simulink model "Assignment2_dcm_2021a"  (R2021a)
settings: Solver=FixedStepAuto  StartTime=0.0  StopTime=inf  FixedStep=1e-3  RelTol=1e-3  EnableMultiTasking=on
undefined symbols (not defined in the file): A0, A1, D0, D1, D10, D11, D12, D13, D2, D3, D4, D5, D6, D7, D8, D9, PTA0, PTA1, PTA2, PTB2, PTB23, PTB3, PTB9, PTC16, PTC17, PTC2, PTC3, PTC4, PTD0, PTD1, PTD2, PTD3
libraries: frdmk64flib x19, etargetslib x10
settings Model: ExtModeTrigDuration=5  Creator=MSI_NB  LastModifiedBy=xxx
settings OptimizationCC: EnhancedBackFolding=on  PassReuseOutputArgsAs=Individual arguments  ZeroExternalMemoryAtStartup=off  ZeroInternalMemoryAtStartup=off  MaxStackSize=64  OptimizeBlockOrder=speed  DifferentSizesBufferReuse=on  OptimizationCustomize=off  EfficientTunableParamExpr=on
settings DebuggingCC: ParameterTunabilityLossMsg=error
settings HardwareCC: ProdBitPerPointer=32  ProdBitPerSizeT=32  ProdBitPerPtrDiffT=32  ProdLargestAtomicInteger=Long  ProdLargestAtomicFloat=Double  ProdWordSize=32  ProdHWDeviceType=ARM Compatible->ARM Cortex
settings SFSimCC: MATLABDynamicMemAlloc=off
settings RTWCC: SystemTargetFile=ert.tlc  HardwareBoard=NXP FRDM-K64F  TLCOptions="-aInlineSetEventsForThisBaseRateFcn=TLC_FALSE -aSuppressMultiTaskScheduler=TLC_FALSE  -aRateBasedStepFcn=0"  TemplateMakefile=ert_default_tmf  Toolchain=GNU Tools for ARM Embedded Processors
settings CodeAppCC: ForceParamTrailComments=on  IgnoreCustomStorageClasses=off  OperatorAnnotations=on  SimulinkDataObjDesc=on  SFDataObjDesc=on  InsertBlockDesc=on
settings ERTTargetCC: ExtModeTransport=4  ExtModeMexFile=sendToCommService

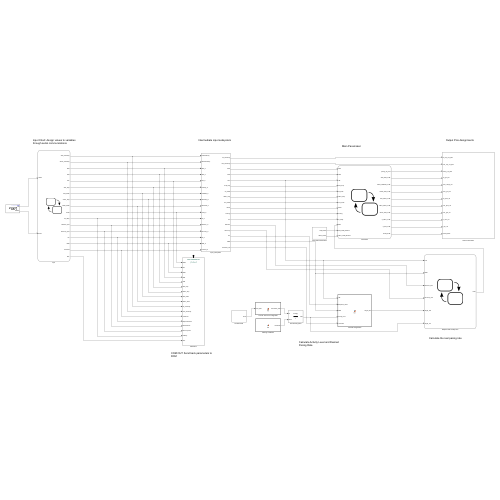
[thumbnail: Simulink's stored preview of the top-level diagram]
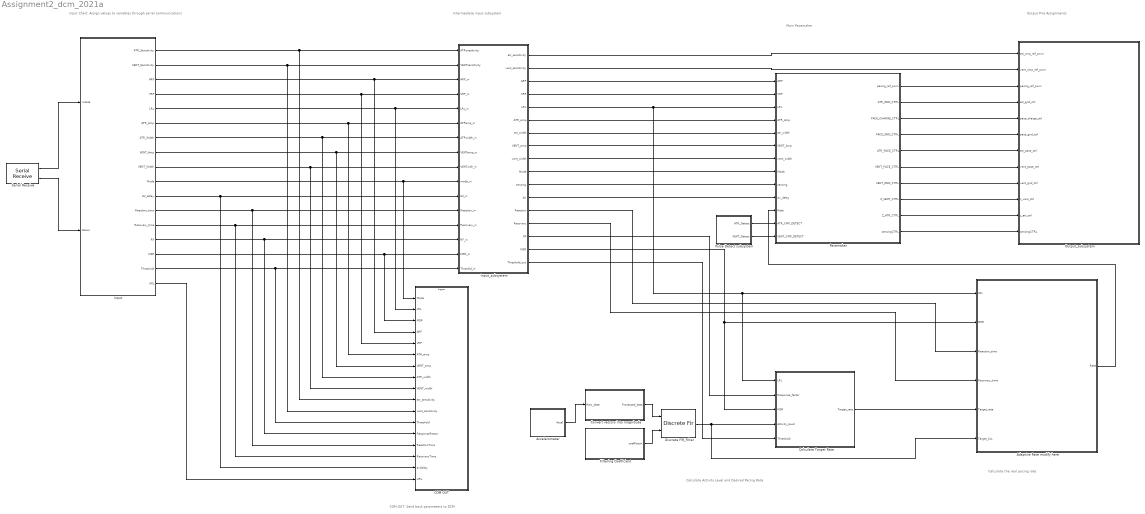
== system Assignment2_dcm_2021a ==
  note: Input Chart: Assign values to variables through serial communications
  note: COM OUT: Send back parameters to DCM
  note: Calculate Activity Level and Desired Pacing Rate
  note: Calculate the real pacing rate
  note: Output Pins Assignments
  note: Main Pacemaker
  note: Intermediate input subsystem
  Accelerometer : Subsystem
  Adaptive Rate modify here : Stateflow chart  TreatAsAtomicUnit=on
      settings: PortSchema="{\"entries\":[{\"content\":{\"sides\":[{\"content\":{\"connectorIds\":[\"In6\",\"In5\",\"In1\",\"In2\",\"In4\",\"In3\"]},\"type\":\"ConnectorPlacement.EquallySpacedRectSide\",\"uuid\":\"39a759a2-6776-4dc2-bf13-d3cf12be31b7\"},{\"content\":{\"connectorIds\":[\"Out1\"],\"side\":\"RIGHT\"},\"type\":\"ConnectorPlacement.EquallySpacedRectSide\",\"uuid\":\"311af287-9fec-40a9-86fa-7b14c4c20eba\"},{\"content\":{\"connectorIds\":[],\"side\":\"TOP\"},\"type\":\"ConnectorPlacement.EquallySpacedRectSide\",\"uuid\":\"bb2111ef-c928-45d1-9471-772f70406d6d\"}]},\"type\":\"ConnectorPlacement.EquallySpacedConnector\",\"uuid\":\"d6adbde0-79db-4fc2-a399-102b42b2f3be\"}],\"packageUris\":[\"http://schema.mathworks.com/mf0/Connector/R2020b\"],\"version\":\"1.0\"}"
  COM OUT : Subsystem  TreatAsAtomicUnit=on
  Calculate Target Rate : MATLAB Function  TreatAsAtomicUnit=on
  Convert vectors into magnitude : MATLAB Function  TreatAsAtomicUnit=on
  Discrete FIR_Filter : DiscreteFir  CoefSource=Input port  Coefficients=[0.05, 0.05, 0.05, 0.05, 0.05, 0.05, 0.05, 0.05, 0.05, 0.05, 0.05, 0.05, 0.05, 0.05, 0.05, 0.05, 0.05, 0.05, 0.05, 0.05]  SampleTime=0.01
      settings: InputPortMap=u0,u1
  Filtering Coefficient : MATLAB Function  TreatAsAtomicUnit=on
  Input : Stateflow chart  TreatAsAtomicUnit=on
      settings: PortSchema="{\"entries\":[{\"content\":{\"sides\":[{\"content\":{\"connectorIds\":[\"In1\",\"In2\"]},\"type\":\"ConnectorPlacement.EquallySpacedRectSide\",\"uuid\":\"ee3611de-e013-4c9d-af16-b184b46b299a\"},{\"content\":{\"connectorIds\":[\"Out6\",\"Out13\",\"Out1\",\"Out2\",\"Out3\",\"Out5\",\"Out7\",\"Out12\",\"Out14\",\"Out8\",\"Out15\",\"Out10\",\"Out11\",\"Out9\",\"Out4\",\"Out17\",\"Out16\"],\"side\":\"RIGHT\"},\"type\":\"ConnectorPlacement.EquallySpacedRectSide\",\"uuid\":\"205a7e36-44cf-418f-ba3c-405c0f3a2ab0\"},{\"content\":{\"connectorIds\":[],\"side\":\"TOP\"},\"type\":\"ConnectorPlacement.EquallySpacedRectSide\",\"uuid\":\"6ab59ebe-c7e2-4512-b8ce-c3a29cac6f4f\"}]},\"type\":\"ConnectorPlacement.EquallySpacedConnector\",\"uuid\":\"f4485e1d-0176-43db-b1e3-40045324a3f2\"}],\"packageUris\":[\"http://schema.mathworks.com/mf0/Connector/R2020b\"],\"version\":\"1.0\"}"
  Input_subsystem : Subsystem
  Output_subsystem : Subsystem
  Pacemaker : Stateflow chart  TreatAsAtomicUnit=on
      settings: PortSchema="{\"entries\":[{\"content\":{\"sides\":[{\"content\":{\"connectorIds\":[\"In1\",\"In10\",\"In6\",\"In8\",\"In11\",\"In7\",\"In12\",\"In3\",\"In5\",\"In13\",\"In9\",\"In2\",\"In4\"]},\"type\":\"ConnectorPlacement.EquallySpacedRectSide\",\"uuid\":\"2ef21990-d536-4d68-b59e-2b2ea3a8851a\"},{\"content\":{\"connectorIds\":[\"Out10\",\"Out1\",\"Out3\",\"Out4\",\"Out2\",\"Out6\",\"Out5\",\"Out7\",\"Out8\",\"Out9\"],\"side\":\"RIGHT\"},\"type\":\"ConnectorPlacement.EquallySpacedRectSide\",\"uuid\":\"f7b17b6e-2681-486a-8f68-6cf7f9b59642\"},{\"content\":{\"connectorIds\":[],\"side\":\"TOP\"},\"type\":\"ConnectorPlacement.EquallySpacedRectSide\",\"uuid\":\"48d212d0-9916-482c-b6c3-a579a81f1368\"},{\"content\":{\"connectorIds\":[],\"side\":\"BOTTOM\"},\"type\":\"ConnectorPlacement.EquallySpacedRectSide\",\"uuid\":\"9c2cce1f-edc0-4859-9c72-07093d7dd567\"}]},\"type\":\"ConnectorPlacement.EquallySpacedConnector\",\"uuid\":\"8d012c1f-5b6f-45ee-bba7-5808d4a194ab\"}],\"packageUris\":[\"http://schema.mathworks.com/mf0/Connector/R2020b\"],\"version\":\"1.0\"}"
  Pulse Detect subsystem : Subsystem
  Serial Receive : frdmk64flib/Serial Receive  SCIModule=0  Baudrate=uint32(9600)  Parity=None  StopBits=1  HardwareFlowControl=None  ByteOrder=LittleEndian  DataType=uint8  DataLength=37  BlockingMode=off  OutputStatus=on  SampleTime=-1
  wires:
  Pulse Detect subsystem/1(ATR_Detect) -> Pacemaker/2(ATR_CMP_DETECT)
  Pulse Detect subsystem/2(VENT_Detect) -> Pacemaker/4(VENT_CMP_DETECT)
  Pacemaker/7(Z_VENT_CTRL) -> Output_subsystem/10(" z_vent_ctrl")
  Pacemaker/8(Z_ATR_CTRL) -> Output_subsystem/11(z_atr_ctrl)
  Pacemaker/5(VENT_GND_CTRL) -> Output_subsystem/9(vent_gnd_ctrl)
  Pacemaker/2(ATR_PACE_CTRL) -> Output_subsystem/7(atr_pace_ctrl)
  Pacemaker/6(VENT_PACE_CTRL) -> Output_subsystem/8(vent_pace_ctrl)
  Pacemaker/4(PACE_GND_CTRL) -> Output_subsystem/6(pace_gnd_ctrl)
  Pacemaker/9(sensingCTRL) -> Output_subsystem/12(sensingCTRL)
  Pacemaker/3(PACE_CHARGE_CTRL) -> Output_subsystem/5(pace_charge_ctrl)
  Pacemaker/1(ATR_GND_CTRL) -> Output_subsystem/4(atr_gnd_ctrl)
  Input_subsystem/4(VRP) -> Pacemaker/10(VRP)
  Input_subsystem/3(ARP) -> Pacemaker/1(ARP)
  Input_subsystem/6(ATR_amp) -> Pacemaker/8(ATR_Amp)
  Input_subsystem/7(atr_width) -> Pacemaker/11(atr_width)
  Input_subsystem/8(VENT_amp) -> Pacemaker/7(VENT_Amp)
  Input_subsystem/9(vent_width) -> Pacemaker/12(vent_width)
  Input_subsystem/10(Mode) -> Pacemaker/3(Mode)
  Adaptive Rate modify here/1(Rate) -> Pacemaker/9(Rate)
  Input_subsystem/13(Reaction) -> Adaptive Rate modify here/1(Reaction_time)
  Input_subsystem/14(Recovery) -> Adaptive Rate modify here/2(Recovery_time)
  Pacemaker/10(pacing_ref_pwm) -> Output_subsystem/3(pacing_ref_pwm)
  Input_subsystem/2(vent_sensitivity) -> Output_subsystem/2(vent_cmp_ref_pwm)
  Input_subsystem/1(atr_sensitivity) -> Output_subsystem/1(atr_cmp_ref_pwm)
  Input_subsystem/11(sensing) -> Pacemaker/5(sensing)
  Convert vectors into magnitude/1(Processed_data) -> Discrete FIR_Filter/1
  Filtering Coefficient/1(coefficient) -> Discrete FIR_Filter/2
  Input_subsystem/16(MSR) -> Adaptive Rate modify here/5(MSR), Calculate Target Rate/3(MSR)
  Calculate Target Rate/1(Target_rate) -> Adaptive Rate modify here/4(Target_rate)
  Input_subsystem/15(RF) -> Calculate Target Rate/2(Response_factor)
  Input_subsystem/5(LRL) -> Adaptive Rate modify here/6(LRL), Calculate Target Rate/1(LRL), Pacemaker/6(LRL)
  Input_subsystem/12(AV) -> Pacemaker/13(av_delay)
  Accelerometer/1(Accel) -> Convert vectors into magnitude/1(Raw_data)
  Serial Receive/1 -> Input/1(rxdata)
  Serial Receive/2 -> Input/2(status)
  Input_subsystem/17(Threshold_out) -> Calculate Target Rate/5(Threshold)
  Discrete FIR_Filter/1 -> Adaptive Rate modify here/3(Target_LVL), Calculate Target Rate/4(Activity_level)
  Input/6(ATR_Sensitivity) -> COM OUT/10(atr_sensitivity), Input_subsystem/1(ATRsnesitivity)
  Input/13(VENT_Sensitivity) -> COM OUT/11(vent_sensitivity), Input_subsystem/2(VENTsensitivity)
  Input/1(ARP) -> COM OUT/4(ARP), Input_subsystem/3(ARP_in)
  Input/2(VRP) -> COM OUT/5(VRP), Input_subsystem/4(VRP_in)
  Input/3(LRL) -> COM OUT/2(LRL), Input_subsystem/5(LRL_in)
  Input/5(ATR_Amp) -> COM OUT/6(ATR_amp), Input_subsystem/6(ATPamp_in)
  Input/7(ATR_Width) -> COM OUT/8(ATR_width), Input_subsystem/7(ATRwidth_in)
  Input/12(VENT_Amp) -> COM OUT/7(VENT_amp), Input_subsystem/8(VENTamp_in)
  Input/14(VENT_Width) -> COM OUT/9(VENT_width), Input_subsystem/9(VENTwith_in)
  Input/8(Mode) -> COM OUT/1(Mode), Input_subsystem/10(mode_in)
  Input/15(AV_delay) -> COM OUT/16(avDelay), Input_subsystem/11(AV_in)
  Input/10(Reaction_time) -> COM OUT/14(ReactionTime), Input_subsystem/12(Reaction_in)
  Input/11(Recovery_time) -> COM OUT/15(RecoveryTime), Input_subsystem/13(Recovery_in)
  Input/9(RF) -> COM OUT/13(ResponseFactor), Input_subsystem/14(RF_in)
  Input/4(MSR) -> COM OUT/3(MSR), Input_subsystem/15(MSR_in)
  Input/17(Threshold) -> COM OUT/12(Threshold), Input_subsystem/16(Threshld_in)
  Input/16(URL) -> COM OUT/17(URL)

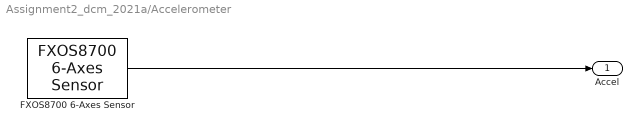
== system Assignment2_dcm_2021a/Accelerometer ==
  FXOS8700 6-Axes Sensor : frdmk64flib/FXOS8700 6-Axes Sensor  Activesensor=Accelerometer only  ODR=800Hz  HybridODR=400Hz  Accelfullrange=-4g to +4g  SampleTime=0.01
  Accel : Outport
  wires:
  FXOS8700 6-Axes Sensor/1 -> Accel/1

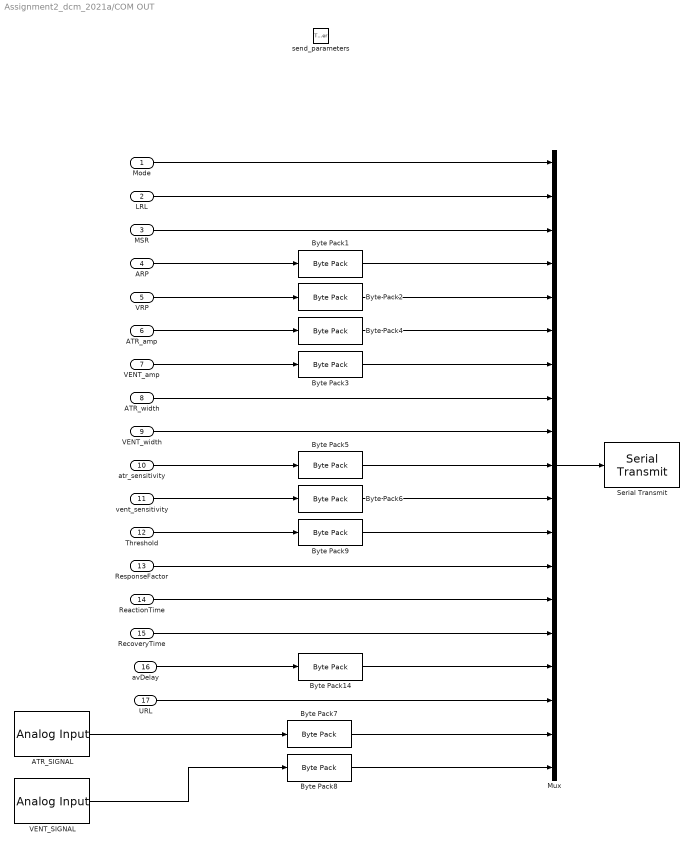
== system Assignment2_dcm_2021a/COM OUT ==
  Mode : Inport  OutDataTypeStr=uint8
  LRL : Inport  Port=2  OutDataTypeStr=uint8
  MSR : Inport  Port=3  OutDataTypeStr=uint8
  ARP : Inport  Port=4  OutDataTypeStr=uint16
  VRP : Inport  Port=5  OutDataTypeStr=uint16
  ATR_amp : Inport  Port=6  OutDataTypeStr=single
  VENT_amp : Inport  Port=7  OutDataTypeStr=single
  ATR_width : Inport  Port=8  OutDataTypeStr=uint8
  VENT_width : Inport  Port=9  OutDataTypeStr=uint8
  atr_sensitivity : Inport  Port=10  OutDataTypeStr=single
  vent_sensitivity : Inport  Port=11  OutDataTypeStr=single
  Threshold : Inport  Port=12  OutDataTypeStr=single
  ResponseFactor : Inport  Port=13  OutDataTypeStr=uint8
  ReactionTime : Inport  Port=14  OutDataTypeStr=uint8
  RecoveryTime : Inport  Port=15  OutDataTypeStr=uint8
  avDelay : Inport  Port=16  OutDataTypeStr=uint16
  URL : Inport  Port=17  OutDataTypeStr=uint8
  send_parameters : TriggerPort  TriggerType=function-call  IsSimulinkFunction=on  FunctionName=send_parameters  VariantControl=(inherit)
  ATR_SIGNAL : frdmk64flib/Analog Input  Whichpin=PTB2 (A0)  SampleTime=-1
  Byte Pack1 : etargetslib/Byte Pack  datatypes={'uint16'}  byteAlign=1
  Byte Pack14 : etargetslib/Byte Pack  datatypes={'uint16'}  byteAlign=1
  Byte Pack2 : etargetslib/Byte Pack  datatypes={'uint16'}  byteAlign=1
  Byte Pack{3..6,9} (5 alike) : etargetslib/Byte Pack  datatypes={'single'}  byteAlign=1
  Byte Pack7 : etargetslib/Byte Pack  datatypes={'double'}  byteAlign=1
  Byte Pack8 : etargetslib/Byte Pack  datatypes={'double'}  byteAlign=1
  Mux : Mux  Inputs=19
  Serial Transmit : frdmk64flib/Serial Transmit  SCIModule=0  Baudrate=uint32(9600)  Parity=None  StopBits=1  HardwareFlowControl=None  ByteOrder=LittleEndian  BlockingMode=on  OutputStatus=off
  VENT_SIGNAL : frdmk64flib/Analog Input  Whichpin=PTB3 (A1)  SampleTime=-1
  wires:
  ReactionTime/1 -> Mux/14
  avDelay/1 -> Byte Pack14/1
  VENT_width/1 -> Mux/9
  vent_sensitivity/1 -> Byte Pack6/1
  MSR/1 -> Mux/3
  VENT_amp/1 -> Byte Pack3/1
  ResponseFactor/1 -> Mux/13
  LRL/1 -> Mux/2
  VRP/1 -> Byte Pack2/1
  Byte Pack5/1 -> Mux/10
  Byte Pack3/1 -> Mux/7
  Byte Pack4/1 -> Mux/6
  ATR_amp/1 -> Byte Pack4/1
  Threshold/1 -> Byte Pack9/1
  atr_sensitivity/1 -> Byte Pack5/1
  Byte Pack2/1 -> Mux/5
  RecoveryTime/1 -> Mux/15
  Byte Pack14/1 -> Mux/16
  Mode/1 -> Mux/1
  Byte Pack9/1 -> Mux/12
  ARP/1 -> Byte Pack1/1
  URL/1 -> Mux/17
  ATR_width/1 -> Mux/8
  Byte Pack6/1 -> Mux/11
  Byte Pack1/1 -> Mux/4
  ATR_SIGNAL/1 -> Byte Pack7/1
  Byte Pack7/1 -> Mux/18
  Byte Pack8/1 -> Mux/19
  VENT_SIGNAL/1 -> Byte Pack8/1
  Mux/1 -> Serial Transmit/1

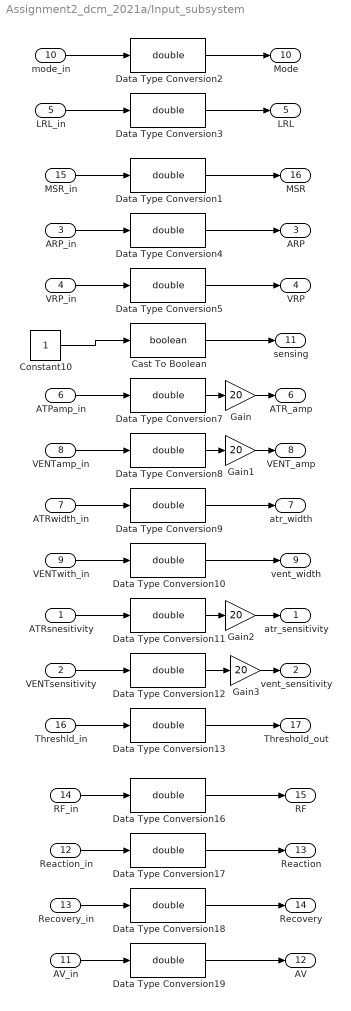
== system Assignment2_dcm_2021a/Input_subsystem ==
  ATRsnesitivity : Inport  Unit=ms
  VENTsensitivity : Inport  Port=2  Unit=ms
  ARP_in : Inport  Port=3  Unit=ms
  VRP_in : Inport  Port=4  Unit=ms
  LRL_in : Inport  Port=5  Unit=ms
  ATPamp_in : Inport  Port=6  Unit=ms
  ATRwidth_in : Inport  Port=7  Unit=ms
  VENTamp_in : Inport  Port=8  Unit=ms
  VENTwith_in : Inport  Port=9  Unit=ms
  mode_in : Inport  Port=10  Unit=ms
  AV_in : Inport  Port=11  Unit=ms
  Reaction_in : Inport  Port=12  Unit=ms
  Recovery_in : Inport  Port=13  Unit=ms
  RF_in : Inport  Port=14  Unit=ms
  MSR_in : Inport  Port=15  Unit=ms
  Threshld_in : Inport  Port=16  Unit=ms
  Cast To Boolean : DataTypeConversion  OutDataTypeStr=boolean
  Constant10 : Constant
  Data Type Conversion{1..5,7..13,16..19} (16 alike) : DataTypeConversion  OutDataTypeStr=double
  Gain{,1..3} (4 alike) : Gain  Gain=20
  atr_sensitivity : Outport
  vent_sensitivity : Outport  Port=2
  ARP : Outport  Port=3
  VRP : Outport  Port=4
  LRL : Outport  Port=5
  ATR_amp : Outport  Port=6
  atr_width : Outport  Port=7
  VENT_amp : Outport  Port=8
  vent_width : Outport  Port=9
  Mode : Outport  Port=10
  sensing : Outport  Port=11
  AV : Outport  Port=12
  Reaction : Outport  Port=13
  Recovery : Outport  Port=14
  RF : Outport  Port=15
  MSR : Outport  Port=16
  Threshold_out : Outport  Port=17
  wires:
  mode_in/1 -> Data Type Conversion2/1
  LRL_in/1 -> Data Type Conversion3/1
  MSR_in/1 -> Data Type Conversion1/1
  ARP_in/1 -> Data Type Conversion4/1
  VRP_in/1 -> Data Type Conversion5/1
  ATPamp_in/1 -> Data Type Conversion7/1
  VENTamp_in/1 -> Data Type Conversion8/1
  ATRwidth_in/1 -> Data Type Conversion9/1
  VENTwith_in/1 -> Data Type Conversion10/1
  ATRsnesitivity/1 -> Data Type Conversion11/1
  VENTsensitivity/1 -> Data Type Conversion12/1
  Threshld_in/1 -> Data Type Conversion13/1
  RF_in/1 -> Data Type Conversion16/1
  Reaction_in/1 -> Data Type Conversion17/1
  Recovery_in/1 -> Data Type Conversion18/1
  AV_in/1 -> Data Type Conversion19/1
  Data Type Conversion3/1 -> LRL/1
  Data Type Conversion1/1 -> MSR/1
  Data Type Conversion4/1 -> ARP/1
  Data Type Conversion5/1 -> VRP/1
  Cast To Boolean/1 -> sensing/1
  Data Type Conversion7/1 -> Gain/1
  Data Type Conversion8/1 -> Gain1/1
  Data Type Conversion9/1 -> atr_width/1
  Data Type Conversion10/1 -> vent_width/1
  Data Type Conversion11/1 -> Gain2/1
  Data Type Conversion12/1 -> Gain3/1
  Data Type Conversion13/1 -> Threshold_out/1
  Data Type Conversion16/1 -> RF/1
  Data Type Conversion17/1 -> Reaction/1
  Data Type Conversion18/1 -> Recovery/1
  Data Type Conversion19/1 -> AV/1
  Data Type Conversion2/1 -> Mode/1
  Constant10/1 -> Cast To Boolean/1
  Gain/1 -> ATR_amp/1
  Gain1/1 -> VENT_amp/1
  Gain2/1 -> atr_sensitivity/1
  Gain3/1 -> vent_sensitivity/1

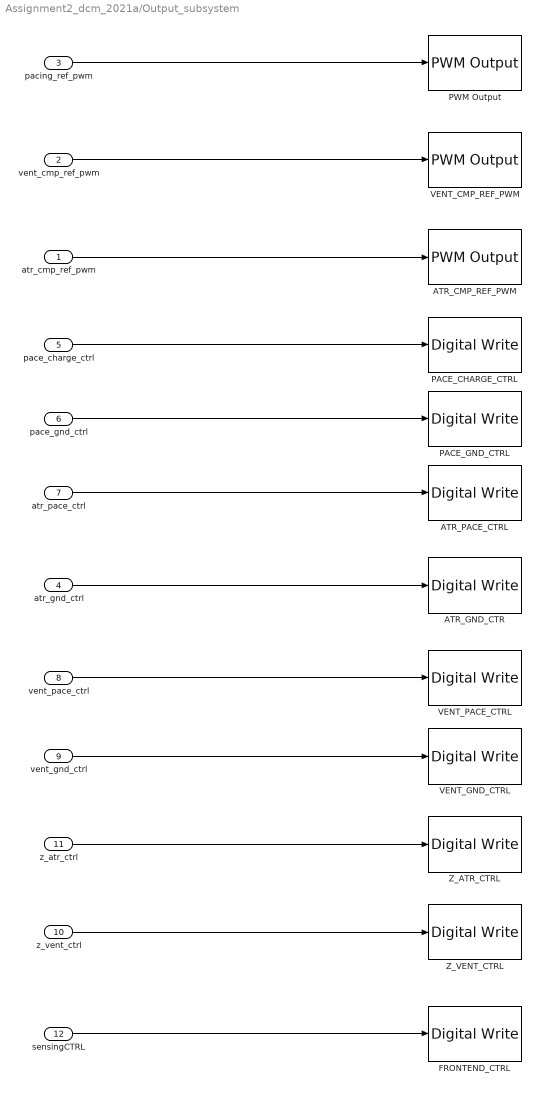
== system Assignment2_dcm_2021a/Output_subsystem ==
  atr_cmp_ref_pwm : Inport
  vent_cmp_ref_pwm : Inport  Port=2
  pacing_ref_pwm : Inport  Port=3
  atr_gnd_ctrl : Inport  Port=4
  pace_charge_ctrl : Inport  Port=5
  pace_gnd_ctrl : Inport  Port=6
  atr_pace_ctrl : Inport  Port=7
  vent_pace_ctrl : Inport  Port=8
  vent_gnd_ctrl : Inport  Port=9
  " z_vent_ctrl" : Inport  Port=10
  z_atr_ctrl : Inport  Port=11
  sensingCTRL : Inport  Port=12
  ATR_CMP_REF_PWM : frdmk64flib/PWM Output  Whichpin=PTC2 (D6)  InitialFrequency=2000  InitialDutyCycle=50
  ATR_GND_CTR : frdmk64flib/Digital Write  Whichpin=PTD2 (D11)
  ATR_PACE_CTRL : frdmk64flib/Digital Write  Whichpin=PTA0 (D8)
  FRONTEND_CTRL : frdmk64flib/Digital Write  Whichpin=PTD1 (D13)
  PACE_CHARGE_CTRL : frdmk64flib/Digital Write  Whichpin=PTB9 (D2)
  PACE_GND_CTRL : frdmk64flib/Digital Write  Whichpin=PTD0 (D10)
  PWM Output : frdmk64flib/PWM Output  Whichpin=PTA2 (D5)  InitialFrequency=2000  InitialDutyCycle=50
  VENT_CMP_REF_PWM : frdmk64flib/PWM Output  Whichpin=PTA1 (D3)  InitialFrequency=2000  InitialDutyCycle=50
  VENT_GND_CTRL : frdmk64flib/Digital Write  Whichpin=PTD3 (D12)
  VENT_PACE_CTRL : frdmk64flib/Digital Write  Whichpin=PTC4 (D9)
  Z_ATR_CTRL : frdmk64flib/Digital Write  Whichpin=PTB23 (D4)
  Z_VENT_CTRL : frdmk64flib/Digital Write  Whichpin=PTC3 (D7)
  wires:
  pace_gnd_ctrl/1 -> PACE_GND_CTRL/1
  atr_pace_ctrl/1 -> ATR_PACE_CTRL/1
  pace_charge_ctrl/1 -> PACE_CHARGE_CTRL/1
  atr_gnd_ctrl/1 -> ATR_GND_CTR/1
  vent_pace_ctrl/1 -> VENT_PACE_CTRL/1
  vent_gnd_ctrl/1 -> VENT_GND_CTRL/1
  z_atr_ctrl/1 -> Z_ATR_CTRL/1
  " z_vent_ctrl"/1 -> Z_VENT_CTRL/1
  sensingCTRL/1 -> FRONTEND_CTRL/1
  pacing_ref_pwm/1 -> PWM Output/1
  vent_cmp_ref_pwm/1 -> VENT_CMP_REF_PWM/1
  atr_cmp_ref_pwm/1 -> ATR_CMP_REF_PWM/1

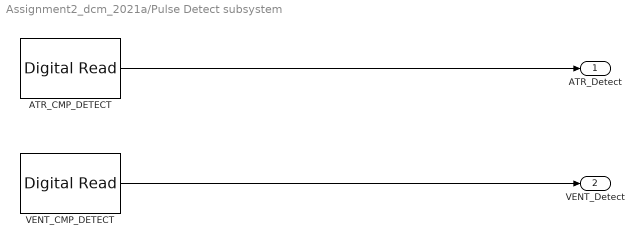
== system Assignment2_dcm_2021a/Pulse Detect subsystem ==
  ATR_CMP_DETECT : frdmk64flib/Digital Read  Whichpin=PTC16 (D0)  SampleTime=-1
  VENT_CMP_DETECT : frdmk64flib/Digital Read  Whichpin=PTC17 (D1)  SampleTime=-1
  ATR_Detect : Outport  OutDataTypeStr=boolean
  VENT_Detect : Outport  Port=2  OutDataTypeStr=boolean
  wires:
  ATR_CMP_DETECT/1 -> ATR_Detect/1
  VENT_CMP_DETECT/1 -> VENT_Detect/1

== stateflow chart Assignment2_dcm_2021a/Input ==
  settings: executeAtInitialization=1
  state SET_PARAM
    entry:
    Mode = rxdata(3);
    LRL = rxdata(4);
    MSR = rxdata(5);
    ARP =  typecast(rxdata(6:7), 'uint16');
    VRP = typecast(rxdata(8:9), 'uint16');
    ATR_Amp = typecast(rxdata(10:13),'single');
    VENT_Amp = typecast(rxdata(14:17),'single');
    ATR_Width = rxdata(18);
    VENT_Width = rxdata(19);
    ATR_Sensitivity = typecast(rxdata(20:23), 'single');
    VENT_Sensitivity = typecast(rxdata(24:27), 'single');
    Threshold = typecast(rxdata(28:31), 'single');
    RF =rxdata(32);
    Reaction_time = rxdata(33);
    Recovery_time =rxdata(34);
    AV_delay = typecast(rxdata(35:36), 'uint16');
    URL = rxdata(37);
  state Initialize
    entry:
    Mode = 1; %select mode:1-10
    LRL = 60; %ppm
    MSR = 160; %ppm
    ARP = 250; %msec
    VRP = 250; %msec
    ATR_Amp = 3.3; %Volt, will convert to dutycycle later
    VENT_Amp = 3.3; %Volt, will convert to dutycycle later
    ATR_Width = 10; %msec
    VENT_Width = 10; %msec
    ATR_Sensitivity = 3; %Volt, will convert to dutycycle later
    VENT_Sensitivity = 3; %Volt, will convert to dutycycle later
    Threshold = 1.1; %Threshold for activity level
    RF = 16; % Response Factor: 1-16
    Reaction_time = 10; %sec
    Recovery_time = 30; %sec
    AV_delay = 150;%msec
    URL = 160; %ppm
  state STANDBY
    %Waiting for COM
  state ECHO_PARAMETERS
    entry:
    send_parameters();
  SET_PARAM -> STANDBY
  (default) -> Initialize
  (junction 115) -> SET_PARAM [order 1] : [rxdata(2) == hex2dec('55')]
  STANDBY -> (junction 118) : [status==0]
  (junction 118) -> (junction 115) : [rxdata(1) == hex2dec('16')]
  Initialize -> STANDBY
  (junction 115) -> ECHO_PARAMETERS [order 2] : [rxdata(2) == hex2dec('22')]
  ECHO_PARAMETERS -> STANDBY
  data: ARP output uint16; VRP output uint16; LRL output uint8; MSR output uint8; ATR_Amp output single; ATR_Sensitivity output single; ATR_Width output uint8; Mode output uint8; RF output uint8; Reaction_time output uint8; Recovery_time output uint8; VENT_Amp output single; VENT_Sensitivity output single; VENT_Width output uint8; AV_delay output uint16; rxdata input uint8; status input uint8 size=[1 1]; URL output uint8; Threshold output single

== stateflow chart Assignment2_dcm_2021a/Pacemaker ==
  state VOO
    state Charging_Discharging
      entry:
      pacing_ref_pwm = VENT_Amp;
      pacing_period = (60000/LRL);
      ATR_PACE_CTRL = false;
      ATR_GND_CTRL = false;
      VENT_PACE_CTRL = false;
      VENT_GND_CTRL = true;
      PACE_GND_CTRL = true;
      Z_ATR_CTRL = false;
      Z_VENT_CTRL = false;
      PACE_CHARGE_CTRL = true;
    state Pacing
      entry:
      PACE_CHARGE_CTRL = false;
      ATR_PACE_CTRL = false;
      ATR_GND_CTRL = false;
      VENT_PACE_CTRL = true;
      VENT_GND_CTRL = false;
      PACE_GND_CTRL = true;
      Z_ATR_CTRL = false;
      Z_VENT_CTRL = false;
    (default) -> VOO.Charging_Discharging
    VOO.Charging_Discharging -> VOO.Pacing : after((pacing_period-vent_width),msec)
    VOO.Pacing -> VOO.Charging_Discharging : after(vent_width,msec)
  state VVI
    state Charging_Discharging
      entry:
      pacing_ref_pwm = VENT_Amp;
      pacing_period = (60000/LRL);
      sensingCTRL = sensing;
      ATR_PACE_CTRL = false;
      ATR_GND_CTRL = false;
      VENT_PACE_CTRL = false;
      VENT_GND_CTRL = true;
      PACE_GND_CTRL = true;
      Z_ATR_CTRL = false;
      Z_VENT_CTRL = false;
      PACE_CHARGE_CTRL = true;
    state Pacing
      entry:
      ATR_PACE_CTRL = false;
      ATR_GND_CTRL = false;
      VENT_PACE_CTRL = true;
      VENT_GND_CTRL = false;
      PACE_GND_CTRL = true;
      Z_ATR_CTRL = false;
      Z_VENT_CTRL = false;
      sensingCTRL = sensing;
    state Sensing_Vent_True
      entry:
      sensingCTRL = true;
    (default) -> VVI.Charging_Discharging
    VVI.Charging_Discharging -> VVI.Pacing [order 2] : after((pacing_period-vent_width),msec){PACE_CHARGE_CTRL = false;}
    VVI.Pacing -> VVI.Charging_Discharging : after(vent_width,msec)
    VVI.Sensing_Vent_True -> VVI.Charging_Discharging : after(vent_width,msec)
    VVI.Charging_Discharging -> VVI.Sensing_Vent_True [order 1] : after((VRP-vent_width),msec)[sensing && (VENT_CMP_DETECT)]
  state VOOR
    state Charging_Discharging
      entry:
      pacing_ref_pwm = VENT_Amp;
      pacing_period = (60000/Rate);
      ATR_PACE_CTRL = false;
      ATR_GND_CTRL = false;
      VENT_PACE_CTRL = false;
      VENT_GND_CTRL = true;
      PACE_GND_CTRL = true;
      Z_ATR_CTRL = false;
      Z_VENT_CTRL = false;
      PACE_CHARGE_CTRL = true;
    state Pacing
      entry:
      PACE_CHARGE_CTRL = false;
      ATR_PACE_CTRL = false;
      ATR_GND_CTRL = false;
      VENT_PACE_CTRL = true;
      VENT_GND_CTRL = false;
      PACE_GND_CTRL = true;
      Z_ATR_CTRL = false;
      Z_VENT_CTRL = false;
    (default) -> VOOR.Charging_Discharging
    VOOR.Charging_Discharging -> VOOR.Pacing : after((pacing_period-vent_width),msec)
    VOOR.Pacing -> VOOR.Charging_Discharging : after(vent_width,msec)
  state Entry_Point
  state VVIR
    state Charging_Discharging
      entry:
      pacing_ref_pwm = VENT_Amp;
      pacing_period = (60000/Rate);
      sensingCTRL = sensing;
      ATR_PACE_CTRL = false;
      ATR_GND_CTRL = false;
      VENT_PACE_CTRL = false;
      VENT_GND_CTRL = true;
      PACE_GND_CTRL = true;
      Z_ATR_CTRL = false;
      Z_VENT_CTRL = false;
      PACE_CHARGE_CTRL = true;
    state Pacing
      entry:
      ATR_PACE_CTRL = false;
      ATR_GND_CTRL = false;
      VENT_PACE_CTRL = true;
      VENT_GND_CTRL = false;
      PACE_GND_CTRL = true;
      Z_ATR_CTRL = false;
      Z_VENT_CTRL = false;
      sensingCTRL = sensing;
    state Sensing_Vent_True
      entry:
      sensingCTRL = true;
    (default) -> VVIR.Charging_Discharging
    VVIR.Charging_Discharging -> VVIR.Pacing [order 2] : after((pacing_period-vent_width),msec){PACE_CHARGE_CTRL = false;}
    VVIR.Pacing -> VVIR.Charging_Discharging : after(vent_width,msec)
    VVIR.Sensing_Vent_True -> VVIR.Charging_Discharging : after(vent_width,msec)
    VVIR.Charging_Discharging -> VVIR.Sensing_Vent_True [order 1] : after((VRP-vent_width),msec)[sensing && (VENT_CMP_DETECT)]
  state AAIR
    state Charging_Discharging1
      entry:
      pacing_ref_pwm = ATR_Amp;
      pacing_period = (60000/Rate);
      sensingCTRL = sensing;
      ATR_PACE_CTRL = false;
      ATR_GND_CTRL = true;
      VENT_PACE_CTRL = false;
      VENT_GND_CTRL = false;
      PACE_GND_CTRL = true;
      Z_ATR_CTRL = false;
      Z_VENT_CTRL = false;
      PACE_CHARGE_CTRL = true;
    state Pacing1
      entry:
      ATR_PACE_CTRL = true;
      ATR_GND_CTRL = false;
      VENT_PACE_CTRL = false;
      VENT_GND_CTRL = false;
      PACE_GND_CTRL = true;
      Z_ATR_CTRL = false;
      Z_VENT_CTRL = false;
      sensingCTRL = sensing;
    state Sensing_ATR
      entry:
      sensingCTRL = true;
    (default) -> AAIR.Charging_Discharging1
    AAIR.Charging_Discharging1 -> AAIR.Pacing1 [order 2] : after((pacing_period-atr_width),msec){PACE_CHARGE_CTRL = false;}
    AAIR.Pacing1 -> AAIR.Charging_Discharging1 : after(atr_width,msec)
    AAIR.Sensing_ATR -> AAIR.Charging_Discharging1 : after(atr_width,msec)
    AAIR.Charging_Discharging1 -> AAIR.Sensing_ATR [order 1] : after((ARP-atr_width),msec)[sensing && (ATR_CMP_DETECT)]
  state AOO
    state Charging_Discharging
      entry:
      pacing_period = (60000/LRL);
      ATR_PACE_CTRL = false;
      VENT_PACE_CTRL = false;
      pacing_ref_pwm = ATR_Amp;
      PACE_CHARGE_CTRL = true;
      PACE_GND_CTRL = true;
      Z_ATR_CTRL = false;
      Z_VENT_CTRL = false;
      ATR_GND_CTRL = true;
      VENT_GND_CTRL = false;
    state Pacing
      entry:
      PACE_CHARGE_CTRL = false;
      PACE_GND_CTRL = true;
      ATR_PACE_CTRL = true;
      ATR_GND_CTRL = false;
      Z_ATR_CTRL = false;
      Z_VENT_CTRL = false;
      VENT_PACE_CTRL = false;
      VENT_GND_CTRL = false;
    (default) -> AOO.Charging_Discharging
    AOO.Charging_Discharging -> AOO.Pacing : after((pacing_period-atr_width),msec)
    AOO.Pacing -> AOO.Charging_Discharging : after(atr_width,msec)
  state AOOR
    state Charging_Discharging
      entry:
      pacing_ref_pwm = ATR_Amp;
      pacing_period = (60000/Rate);
      ATR_PACE_CTRL = false;
      ATR_GND_CTRL = true;
      VENT_PACE_CTRL = false;
      VENT_GND_CTRL = false;
      PACE_GND_CTRL = true;
      Z_ATR_CTRL = false;
      Z_VENT_CTRL = false;
      PACE_CHARGE_CTRL = true;
    state Pacing
      entry:
      PACE_CHARGE_CTRL = false;
      ATR_PACE_CTRL = true;
      ATR_GND_CTRL = false;
      VENT_PACE_CTRL = false;
      VENT_GND_CTRL = false;
      PACE_GND_CTRL = true;
      Z_ATR_CTRL = false;
      Z_VENT_CTRL = false;
    (default) -> AOOR.Charging_Discharging
    AOOR.Charging_Discharging -> AOOR.Pacing : after((pacing_period - atr_width),msec)
    AOOR.Pacing -> AOOR.Charging_Discharging : after(atr_width,msec)
  state AAI
    state Charging_Discharging1
      entry:
      pacing_ref_pwm = ATR_Amp;
      pacing_period = (60000/LRL);
      sensingCTRL = sensing;
      ATR_PACE_CTRL = false;
      ATR_GND_CTRL = true;
      VENT_PACE_CTRL = false;
      VENT_GND_CTRL = false;
      PACE_GND_CTRL = true;
      Z_ATR_CTRL = false;
      Z_VENT_CTRL = false;
      PACE_CHARGE_CTRL = true;
    state Pacing1
      entry:
      ATR_PACE_CTRL = true;
      ATR_GND_CTRL = false;
      VENT_PACE_CTRL = false;
      VENT_GND_CTRL = false;
      PACE_GND_CTRL = true;
      Z_ATR_CTRL = false;
      Z_VENT_CTRL = false;
      sensingCTRL = sensing;
    state Sensing_ATR
      entry:
      sensingCTRL = true;
    (default) -> AAI.Charging_Discharging1
    AAI.Charging_Discharging1 -> AAI.Pacing1 [order 2] : after((pacing_period-vent_width),msec){PACE_CHARGE_CTRL = false;}
    AAI.Pacing1 -> AAI.Charging_Discharging1 : after(vent_width,msec)
    AAI.Sensing_ATR -> AAI.Charging_Discharging1 : after(vent_width,msec)
    AAI.Charging_Discharging1 -> AAI.Sensing_ATR [order 1] : after((ARP-vent_width),msec)[sensing && (ATR_CMP_DETECT)]
  state DOO
    state Charging_Discharging_A
      entry:
      pacing_ref_pwm = ATR_Amp;
      pacing_period = (60000/LRL);
      ATR_PACE_CTRL = false;
      ATR_GND_CTRL = true;
      VENT_PACE_CTRL = false;
      VENT_GND_CTRL = false;
      PACE_GND_CTRL = true;
      Z_ATR_CTRL = false;
      Z_VENT_CTRL = false;
      PACE_CHARGE_CTRL = true;
    state Pacing_Atrial
      entry:
      PACE_CHARGE_CTRL = false;
      ATR_PACE_CTRL = true;
      ATR_GND_CTRL = false;
      VENT_PACE_CTRL = false;
      VENT_GND_CTRL = false;
      PACE_GND_CTRL = true;
      Z_ATR_CTRL = false;
      Z_VENT_CTRL = false;
    state ChargingV_DischargingA
      entry:
      %%Discharge Atrial
      PACE_GND_CTRL = true;
      VENT_PACE_CTRL = false;
      Z_ATR_CTRL = false;
      Z_VENT_CTRL = false;
      ATR_PACE_CTRL = false;
      ATR_GND_CTRL = true;
      VENT_GND_CTRL = false;
      %%Charge Ventricle
      pacing_ref_pwm = VENT_Amp;
      pacing_period = (60000/LRL);
      ATR_PACE_CTRL = false;
      VENT_PACE_CTRL = false;
      PACE_CHARGE_CTRL = true;
    state ChargingA_DischargingV
      entry:
      %%Discharge Atrial
      PACE_GND_CTRL = true;
      VENT_PACE_CTRL = false;
      Z_ATR_CTRL = false;
      Z_VENT_CTRL = false;
      ATR_PACE_CTRL = false;
      ATR_GND_CTRL = false;
      VENT_GND_CTRL = true;
      %%Charge Ventricle
      pacing_ref_pwm = ATR_Amp;
      pacing_period = (60000/LRL);
      ATR_PACE_CTRL = false;
      VENT_PACE_CTRL = false;
      PACE_CHARGE_CTRL = true;
    state Pacing_Ventricle
      entry:
      PACE_CHARGE_CTRL = false;
      ATR_PACE_CTRL = false;
      ATR_GND_CTRL = false;
      VENT_PACE_CTRL = true;
      VENT_GND_CTRL = false;
      PACE_GND_CTRL = true;
      Z_ATR_CTRL = false;
      Z_VENT_CTRL = false;
    (default) -> DOO.Charging_Discharging_A
    DOO.Charging_Discharging_A -> DOO.Pacing_Atrial : after((pacing_period-atr_width),msec)
    DOO.Pacing_Atrial -> DOO.ChargingV_DischargingA : after(atr_width,msec)
    DOO.ChargingA_DischargingV -> DOO.Pacing_Atrial : after((pacing_period-av_delay-vent_width),msec)
    DOO.ChargingV_DischargingA -> DOO.Pacing_Ventricle : after((av_delay-atr_width),msec)
    DOO.Pacing_Ventricle -> DOO.ChargingA_DischargingV : after(vent_width,msec)
  state DOOR
    state Charging_Discharging_A
      entry:
      pacing_ref_pwm = ATR_Amp;
      pacing_period = (60000/Rate);
      ATR_PACE_CTRL = false;
      ATR_GND_CTRL = true;
      VENT_PACE_CTRL = false;
      VENT_GND_CTRL = false;
      PACE_GND_CTRL = true;
      Z_ATR_CTRL = false;
      Z_VENT_CTRL = false;
      PACE_CHARGE_CTRL = true;
    state Pacing_Atrial
      entry:
      PACE_CHARGE_CTRL = false;
      ATR_PACE_CTRL = true;
      ATR_GND_CTRL = false;
      VENT_PACE_CTRL = false;
      VENT_GND_CTRL = false;
      PACE_GND_CTRL = true;
      Z_ATR_CTRL = false;
      Z_VENT_CTRL = false;
    state ChargingV_DischargingA
      entry:
      %%Discharge Atrial
      PACE_GND_CTRL = true;
      VENT_PACE_CTRL = false;
      Z_ATR_CTRL = false;
      Z_VENT_CTRL = false;
      ATR_PACE_CTRL = false;
      ATR_GND_CTRL = true;
      VENT_GND_CTRL = false;
      %%Charge Ventricle
      pacing_ref_pwm = VENT_Amp;
      pacing_period = (60000/Rate);
      ATR_PACE_CTRL = false;
      VENT_PACE_CTRL = false;
      PACE_CHARGE_CTRL = true;
    state ChargingA_DischargingV
      entry:
      %%Discharge Atrial
      PACE_GND_CTRL = true;
      VENT_PACE_CTRL = false;
      Z_ATR_CTRL = false;
      Z_VENT_CTRL = false;
      ATR_PACE_CTRL = false;
      ATR_GND_CTRL = false;
      VENT_GND_CTRL = true;
      %%Charge Ventricle
      pacing_ref_pwm = ATR_Amp;
      pacing_period = (60000/Rate);
      ATR_PACE_CTRL = false;
      VENT_PACE_CTRL = false;
      PACE_CHARGE_CTRL = true;
    state Pacing_Ventricle
      entry:
      PACE_CHARGE_CTRL = false;
      ATR_PACE_CTRL = false;
      ATR_GND_CTRL = false;
      VENT_PACE_CTRL = true;
      VENT_GND_CTRL = false;
      PACE_GND_CTRL = true;
      Z_ATR_CTRL = false;
      Z_VENT_CTRL = false;
    (default) -> DOOR.Charging_Discharging_A
    DOOR.Charging_Discharging_A -> DOOR.Pacing_Atrial : after((pacing_period-atr_width),msec)
    DOOR.Pacing_Atrial -> DOOR.ChargingV_DischargingA : after(atr_width,msec)
    DOOR.ChargingA_DischargingV -> DOOR.Pacing_Atrial : after((pacing_period-av_delay-vent_width),msec)
    DOOR.ChargingV_DischargingA -> DOOR.Pacing_Ventricle : after((av_delay-atr_width),msec)
    DOOR.Pacing_Ventricle -> DOOR.ChargingA_DischargingV : after(vent_width,msec)
  VOO -> Entry_Point : [Mode ~= 3]
  VVI -> Entry_Point : [Mode ~= 7]
  Entry_Point -> VOO [order 3] : [Mode == 3]
  Entry_Point -> VVI [order 4] : [Mode == 7]
  (default) -> Entry_Point
  Entry_Point -> VOOR [order 6] : [Mode == 4]
  VOOR -> Entry_Point : [Mode ~= 4]
  Entry_Point -> VVIR [order 8] : [Mode == 8]
  VVIR -> Entry_Point : [Mode ~= 8]
  Entry_Point -> AAIR [order 7] : [Mode == 6]
  Entry_Point -> AOO [order 1] : [Mode == 1]
  AAIR -> Entry_Point : [Mode ~= 6]
  AOO -> Entry_Point : [Mode ~= 1]
  Entry_Point -> AAI [order 2] : [Mode == 5]
  Entry_Point -> AOOR [order 5] : [Mode == 2]
  AOOR -> Entry_Point : [Mode ~= 2]
  Entry_Point -> DOO [order 9] : [Mode == 9]
  DOO -> Entry_Point : [Mode ~= 9]
  DOOR -> Entry_Point : [Mode ~= 10]
  Entry_Point -> DOOR [order 10] : [Mode == 10]
  AAI -> Entry_Point : [Mode ~= 5]
  data: ATR_GND_CTRL output boolean; ATR_PACE_CTRL output boolean; PACE_CHARGE_CTRL output boolean; PACE_GND_CTRL output boolean; VENT_GND_CTRL output boolean; VENT_PACE_CTRL output boolean; Z_VENT_CTRL output boolean; Z_ATR_CTRL output boolean; ARP input; ATR_CMP_DETECT input; Mode input; VENT_CMP_DETECT input; sensing input; sensingCTRL output; LRL input; pacing_ref_pwm output; VENT_Amp input; pacing_period local; ATR_Amp input; Rate input; VRP input; atr_width input; vent_width input; av_delay input

== matlab function Assignment2_dcm_2021a/Filtering Coefficient ==
  data: coefficient output double
%This function creates the coefficient for the signal filter.
%It generates an array of all ones, it takes each 200 samples and calculate
%the average.
function coefficient = fcn()
coefficient = (1/200)*ones(1,200);

== matlab function Assignment2_dcm_2021a/Calculate Target Rate ==
  data: Target_rate output double; LRL input; Response_factor input; MSR input; Activity_level input; Threshold input
%This function calculates the target pacing rate corresponding to the activity
%level.
function Target_rate = fcn(LRL, Response_factor, MSR, Activity_level, Threshold)

      if(Activity_level > Threshold)
             
         x1 = LRL + Activity_level*Response_factor;
         if(x1 > MSR)
             Target_rate = MSR;
         else
             Target_rate = x1;
         end
      else
          Target_rate = LRL;
      end

== stateflow chart Assignment2_dcm_2021a/Adaptive Rate modify here ==
  state Entry_Only
    entry:
    %Default Values
    CMP_LVL = 0;
    Rate=LRL;
  state Stand_by
    %Decide whether to increase the Rate or decrease the Rate
  state INCREASE
    entry:
    if (Rate < Target_rate)
    Rate = Rate + ((MSR - LRL)/Reaction_time);
    end
    if(Rate > Target_rate)
    Rate = Target_rate;
    end
  state DECREASE
    entry:
    if (Rate > Target_rate)
    Rate = Rate - ((MSR - LRL)/Recovery_time);
    end
    if(Rate < Target_rate)
    Rate = Target_rate;
    end
  (default) -> Entry_Only
  Entry_Only -> Stand_by
  Stand_by -> INCREASE [order 1] : [Target_LVL > CMP_LVL]{CMP_LVL = Target_LVL;}
  INCREASE -> Stand_by [order 1] : [Target_LVL ~= CMP_LVL]
  DECREASE -> Stand_by [order 1] : [Target_LVL ~= CMP_LVL]
  Stand_by -> DECREASE [order 2] : [Target_LVL < CMP_LVL]{CMP_LVL = Target_LVL;}
  DECREASE -> DECREASE [order 2] : after(1000,msec)[Target_LVL == CMP_LVL]
  INCREASE -> INCREASE [order 2] : after(1000,msec)[Target_LVL == CMP_LVL]
  data: Reaction_time input; Recovery_time input; Target_LVL input; Target_rate input; CMP_LVL local; MSR input; LRL input; Rate output

== matlab function Assignment2_dcm_2021a/Convert vectors into magnitude ==
  data: Raw_data input; Processed_data output
%This function calculate the magnitude of the input-3dimentional-vector input
function Processed_data = fcn(Raw_data)

         Processed_data = sqrt((Raw_data(1))^2+(Raw_data(2))^2+(Raw_data(3))^2);
